simulink library "veh_vehicle_model_lib"  (R2016b)
settings: Solver=ode45  StartTime=0.0  StopTime=10.0  RelTol=1e-3  EnableMultiTasking=on
undefined symbols (not defined in the file): abp_impeller_speed2pwm, tun_sim_cg_error
libraries: util_generic_model_lib x2, epson_imu_model_lib x1
settings Model: Creator=jfusco1  LastModifiedBy=jfusco1
settings DataIOCC: LimitDataPoints=on  SaveFormat=Array
settings OptimizationCC: LifeSpan=inf
settings DebuggingCC: SolverPrmCheckMsg=warning  AllowSymbolicDim=off  SFUnexpectedBacktrackingDiag=warning  SFNoUnconditionalDefaultTransitionDiag=warning  SFExecutionAtInitializationDiag=none
settings HardwareCC: ProdBitPerPointer=32  ProdBitPerSizeT=32  ProdBitPerPtrDiffT=32  ProdLargestAtomicFloat=None  ProdIntDivRoundTo=Undefined  ProdEndianess=Unspecified  ProdWordSize=32  ProdHWDeviceType=32-bit Generic
settings ModelReferenceCC: PropagateSignalLabelsOutOfModel=off
settings GRTTargetCC: TargetLangStandard=C89/C90 (ANSI)  GeneratePreprocessorConditionals=Disable all
settings ConfigComp: CovMetricSettings=dw  CovHtmlReporting=on  CovSaveCumulativeToWorkspaceVar=on  CovSaveSingleToWorkspaceVar=on  CovExternalEMLEnable=off  CovSFcnEnable=off

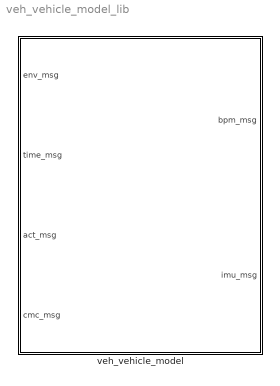
== system veh_vehicle_model_lib ==
  veh_vehicle_model : Subsystem

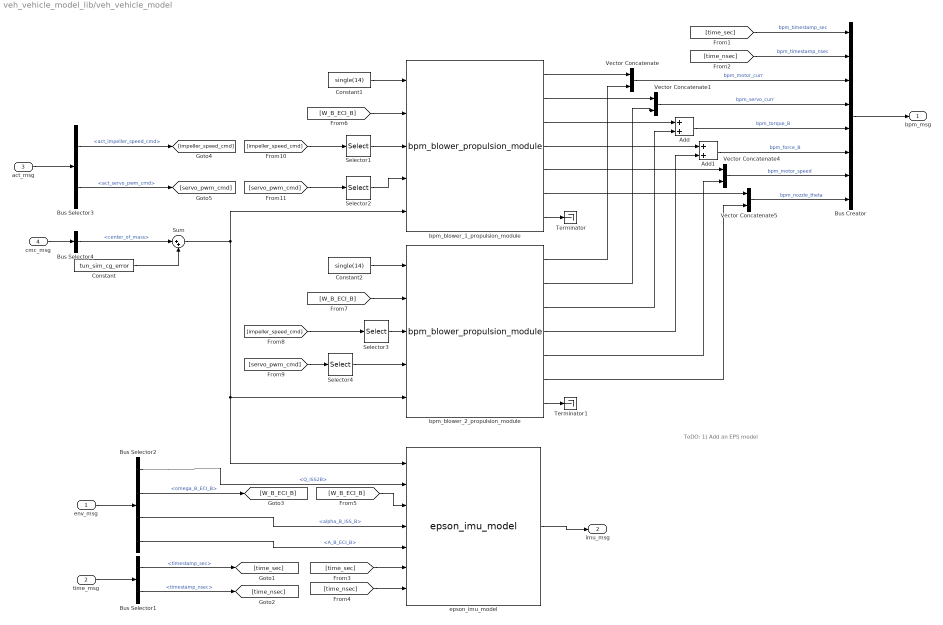
== system veh_vehicle_model_lib/veh_vehicle_model ==
  note: ToDO:
      | 1) Add an EPS model
  env_msg : Inport  OutDataTypeStr=Bus: env_msg
  time_msg : Inport  Port=2
  act_msg : Inport  Port=3
  cmc_msg : Inport  Port=4  OutDataTypeStr=Bus: cmc_msg
  Add : Sum
  Add1 : Sum
  Bus Creator : BusCreator  Inputs=8  OutDataTypeStr=Bus: bpm_msg  NonVirtualBus=on
      settings: InheritFromInputs=off
  Bus Selector1 : BusSelector  OutputSignals=timestamp_sec,timestamp_nsec
  Bus Selector2 : BusSelector  OutputSignals=Q_ISS2B,omega_B_ECI_B,alpha_B_ISS_B,A_B_ECI_B
  Bus Selector3 : BusSelector  OutputSignals=act_impeller_speed_cmd,act_servo_pwm_cmd
  Bus Selector4 : BusSelector  OutputSignals=center_of_mass
  Constant : Constant  Value=tun_sim_cg_error
  Constant1 : Constant  Value=single(14)
  Constant2 : Constant  Value=single(14)
  Selector1 : Selector  InputPortWidth=2  IndexOptions=Index vector (dialog)  Indices=1  OutputSizes=1
      settings: AttributesFormatString=|
      | Input Width: %<InputPortWidth>
      | Selection: %<Indices>
  Selector2 : Selector  InputPortWidth=12  IndexOptions=Index vector (dialog)  Indices=1:6  OutputSizes=1
      settings: AttributesFormatString=|
      | Input Width: %<InputPortWidth>
      | Selection: %<Indices>
  Selector3 : Selector  InputPortWidth=2  IndexOptions=Index vector (dialog)  Indices=2  OutputSizes=1
      settings: AttributesFormatString=|
      | Input Width: %<InputPortWidth>
      | Selection: %<Indices>
  Selector4 : Selector  InputPortWidth=12  IndexOptions=Index vector (dialog)  Indices=7:12  OutputSizes=1
      settings: AttributesFormatString=|
      | Input Width: %<InputPortWidth>
      | Selection: %<Indices>
  Sum : Sum  Inputs=|++
  Terminator : Terminator
  Terminator1 : Terminator
  Vector Concatenate{,1,4..5} (4 alike) : Concatenate
  bpm_blower_1_propulsion_module : util_generic_model_lib/bpm_blower_propulsion_module  s_ctl_ts=bpm_servo_ctl_ts  s_ctl_pwm2angle=bpm_servo_pwm2angle  s_ctl_pwm2angle_bias=bpm_servo_pwm2angle_bias  s_ctl_kp=bpm_servo_ctl_kp  s_ctl_ki=bpm_servo_ctl_ki  s_ctl_kd=bpm_servo_ctl_kd  s_ctl_filt_n=bpm_servo_ctl_filt_n  s_ctl_max_volt=bpm_servo_max_voltage  s_motor_k=bpm_servo_motor_k  s_motor_r=bpm_servo_motor_r  s_motor_friction_coeff=bpm_servo_motor_friction_coeff  s_motor_gear_ratio=bpm_servo_motor_gear_ratio  s_motor_gear_box_inertia=bpm_servo_motor_gear_box_inertia  servo_max_theta=bpm_servo_max_theta  servo_min_theta=bpm_servo_min_theta  servo_backlash_deadband=bpm_servo_motor_backlash_deadband  P_nozzle_B_B=abp_PM1_P_nozzle_B_B  P_nozzle_B_B_offset=bpm_PM1_P_nozzle_B_B_error  nozzle_orientation_B=abp_PM1_nozzle_orientations  nozzle_orientation_offset=bpm_PM1_Q_nozzle2misaligned  noz_cd=abp_PM1_discharge_coeff  noz_cd_error=bpm_PM1_nozzle_discharge_coeff_error  noz_width=abp_PM1_nozzle_widths  noz_min_theta=abp_nozzle_min_open_angle  noz_intake_height=abp_nozzle_intake_height  noz_flap_length=abp_nozzle_flap_length  noz_flap_count=abp_nozzle_flap_count  noz_gear_ratio=abp_nozzle_gear_ratio  noz_thrust_noise=bpm_PM1_nozzle_thrust_noise_1s  noz_thrust_noise_feedback=bpm_PM1_nozzle_noise_feedback_gain  noz_randn_seed=bpm_PM1_randn_noise_seed  i_ctl_ts=bpm_imp_ctl_ts  i_ctl_pwm2speed=1/abp_impeller_speed2pwm  i_ctl_cmd_filt_num=bpm_imp_cmd_filt_num  i_ctl_cmd_filt_den=bpm_imp_cmd_filt_den  i_ctl_speed_filt_num=bpm_imp_speed_filt_num  i_ctl_speed_filt_den=bpm_imp_speed_filt_den  i_ctl_kp=bpm_imp_ctl_kp  i_ctl_ki=bpm_imp_ctl_ki  i_ctl_kd=bpm_imp_ctl_kd  i_ctl_filt_n=bpm_imp_ctl_filt_n  i_ctl_max_volt=bpm_imp_max_voltage  i_motor_kn=bpm_imp_motor_speed_k  i_motor_r=bpm_imp_motor_r  i_motor_kt=bpm_imp_motor_torque_k  i_motor_friction_coeff=bpm_imp_motor_friction_coeff  imp_unit_vec_B=abp_pm1_impeller_orientation  imp_unit_vec_B_offset=bmp_PM1_impeller_orientation_error  imp_zero_thrust_area=abp_pm1_zero_thrust_area  imp_zero_thrust_area_error=bpm_PM1_zero_thrust_area_error  imp_diameter=abp_impeller_diameter  imp_cdp_lookup=bpm_lookup_Cdp_data  imp_area_lookup=bpm_lookup_totalarea_breakpoints  imp_inertia=bpm_impeller_inertia  imp_inertia_error=bpm_impeller_inertia_error  imp_init_speed=bpm_impeller_init_speed  sens_sf=bpm_sensor_sf  sens_sigma_u=bpm_sensor_sigma_u  sens_sigma_v=bpm_sensor_sigma_v  sens_rand_seed=bpm_sensor_rand_seed  sens_resolution=bpm_sensor_resolution  sens_max=bpm_sensor_max  sens_min=bpm_sensor_min  sens_delay=bpm_sensor_delay  P_CG_B_B_error=abp_P_CG_B_B_error  const_air_den=const_air_density  sim_step_size=astrobee_time_step_size  noise_on_flag=tun_bpm_noise_on_flag
  bpm_blower_2_propulsion_module : util_generic_model_lib/bpm_blower_propulsion_module  s_ctl_ts=bpm_servo_ctl_ts  s_ctl_pwm2angle=bpm_servo_pwm2angle  s_ctl_pwm2angle_bias=bpm_servo_pwm2angle_bias  s_ctl_kp=bpm_servo_ctl_kp  s_ctl_ki=bpm_servo_ctl_ki  s_ctl_kd=bpm_servo_ctl_kd  s_ctl_filt_n=bpm_servo_ctl_filt_n  s_ctl_max_volt=bpm_servo_max_voltage  s_motor_k=bpm_servo_motor_k  s_motor_r=bpm_servo_motor_r  s_motor_friction_coeff=bpm_servo_motor_friction_coeff  s_motor_gear_ratio=bpm_servo_motor_gear_ratio  s_motor_gear_box_inertia=bpm_servo_motor_gear_box_inertia  servo_max_theta=bpm_servo_max_theta  servo_min_theta=bpm_servo_min_theta  servo_backlash_deadband=bpm_servo_motor_backlash_deadband  P_nozzle_B_B=abp_PM2_P_nozzle_B_B  P_nozzle_B_B_offset=bpm_PM2_P_nozzle_B_B_error  nozzle_orientation_B=abp_PM2_nozzle_orientations  nozzle_orientation_offset=bpm_PM2_Q_nozzle2misaligned  noz_cd=abp_PM2_discharge_coeff  noz_cd_error=bpm_PM2_nozzle_discharge_coeff_error  noz_width=abp_PM2_nozzle_widths  noz_min_theta=abp_nozzle_min_open_angle  noz_intake_height=abp_nozzle_intake_height  noz_flap_length=abp_nozzle_flap_length  noz_flap_count=abp_nozzle_flap_count  noz_gear_ratio=abp_nozzle_gear_ratio  noz_thrust_noise=bpm_PM2_nozzle_thrust_noise_1s  noz_thrust_noise_feedback=bpm_PM2_nozzle_noise_feedback_gain  noz_randn_seed=bpm_PM2_randn_noise_seed  i_ctl_ts=bpm_imp_ctl_ts  i_ctl_pwm2speed=1/abp_impeller_speed2pwm  i_ctl_cmd_filt_num=bpm_imp_cmd_filt_num  i_ctl_cmd_filt_den=bpm_imp_cmd_filt_den  i_ctl_speed_filt_num=bpm_imp_speed_filt_num  i_ctl_speed_filt_den=bpm_imp_speed_filt_den  i_ctl_kp=bpm_imp_ctl_kp  i_ctl_ki=bpm_imp_ctl_ki  i_ctl_kd=bpm_imp_ctl_kd  i_ctl_filt_n=bpm_imp_ctl_filt_n  i_ctl_max_volt=bpm_imp_max_voltage  i_motor_kn=bpm_imp_motor_speed_k  i_motor_r=bpm_imp_motor_r  i_motor_kt=bpm_imp_motor_torque_k  i_motor_friction_coeff=bpm_imp_motor_friction_coeff  imp_unit_vec_B=abp_pm2_impeller_orientation  imp_unit_vec_B_offset=bmp_PM2_impeller_orientation_error  imp_zero_thrust_area=abp_pm2_zero_thrust_area  imp_zero_thrust_area_error=bpm_PM2_zero_thrust_area_error  imp_diameter=abp_impeller_diameter  imp_cdp_lookup=bpm_lookup_Cdp_data  imp_area_lookup=bpm_lookup_totalarea_breakpoints  imp_inertia=bpm_impeller_inertia  imp_inertia_error=bpm_impeller_inertia_error  imp_init_speed=bpm_impeller_init_speed  sens_sf=bpm_sensor_sf  sens_sigma_u=bpm_sensor_sigma_u  sens_sigma_v=bpm_sensor_sigma_v  sens_rand_seed=bpm_sensor_rand_seed  sens_resolution=bpm_sensor_resolution  sens_max=bpm_sensor_max  sens_min=bpm_sensor_min  sens_delay=bpm_sensor_delay  P_CG_B_B_error=abp_P_CG_B_B_error  const_air_den=const_air_density  sim_step_size=astrobee_time_step_size  noise_on_flag=tun_bpm_noise_on_flag
  epson_imu_model : epson_imu_model_lib/epson_imu_model
  bpm_msg : Outport
  imu_msg : Outport  Port=2
  wires:
  Selector4/1 -> bpm_blower_2_propulsion_module/4
  Selector3/1 -> bpm_blower_2_propulsion_module/3
  Selector2/1 -> bpm_blower_1_propulsion_module/4
  Selector1/1 -> bpm_blower_1_propulsion_module/3
  epson_imu_model/1 -> imu_msg/1
  env_msg/1 -> Bus Selector2/1
  Bus Selector2/2 -> [W_B_ECI_B]  "<omega_B_ECI_B>"
  Bus Selector3/2 -> [servo_pwm_cmd]  "<act_servo_pwm_cmd>"
  Bus Selector3/1 -> [impeller_speed_cmd]  "<act_impeller_speed_cmd>"
  act_msg/1 -> Bus Selector3/1
  time_msg/1 -> Bus Selector1/1
  Bus Selector1/2 -> [time_nsec]  "<timestamp_nsec>"
  Bus Selector1/1 -> [time_sec]  "<timestamp_sec>"
  [time_sec] -> Bus Creator/1  "bpm_timestamp_sec"
  [time_nsec] -> Bus Creator/2  "bpm_timestamp_nsec"
  Vector Concatenate5/1 -> Bus Creator/8  "bpm_nozzle_theta"
  Vector Concatenate4/1 -> Bus Creator/7  "bpm_motor_speed"
  Add/1 -> Bus Creator/5  "bpm_torque_B"
  Add1/1 -> Bus Creator/6  "bpm_force_B"
  Vector Concatenate1/1 -> Bus Creator/4  "bpm_servo_curr"
  Vector Concatenate/1 -> Bus Creator/3  "bpm_motor_curr"
  Bus Creator/1 -> bpm_msg/1
  Constant1/1 -> bpm_blower_1_propulsion_module/1
  Constant2/1 -> bpm_blower_2_propulsion_module/1
  [W_B_ECI_B] -> bpm_blower_1_propulsion_module/2
  [W_B_ECI_B] -> bpm_blower_2_propulsion_module/2
  [servo_pwm_cmd] -> Selector4/1
  [impeller_speed_cmd] -> Selector3/1
  [servo_pwm_cmd] -> Selector2/1
  [impeller_speed_cmd] -> Selector1/1
  bpm_blower_1_propulsion_module/1 -> Vector Concatenate/1
  bpm_blower_1_propulsion_module/2 -> Vector Concatenate1/1
  bpm_blower_1_propulsion_module/3 -> Add/1
  bpm_blower_1_propulsion_module/4 -> Add1/1
  bpm_blower_1_propulsion_module/5 -> Vector Concatenate4/1
  bpm_blower_1_propulsion_module/6 -> Vector Concatenate5/1
  bpm_blower_2_propulsion_module/1 -> Vector Concatenate/2
  bpm_blower_1_propulsion_module/7 -> Terminator/1
  bpm_blower_2_propulsion_module/7 -> Terminator1/1
  bpm_blower_2_propulsion_module/2 -> Vector Concatenate1/2
  bpm_blower_2_propulsion_module/3 -> Add/2
  bpm_blower_2_propulsion_module/4 -> Add1/2
  bpm_blower_2_propulsion_module/5 -> Vector Concatenate4/2
  bpm_blower_2_propulsion_module/6 -> Vector Concatenate5/2
  [W_B_ECI_B] -> epson_imu_model/3
  Bus Selector2/3 -> epson_imu_model/4  "<alpha_B_ISS_B>"
  Bus Selector2/4 -> epson_imu_model/5  "<A_B_ECI_B>"
  [time_sec] -> epson_imu_model/6
  [time_nsec] -> epson_imu_model/7
  Bus Selector2/1 -> epson_imu_model/2  "<Q_ISS2B>"
  cmc_msg/1 -> Bus Selector4/1
  Sum/1 -> epson_imu_model/1, bpm_blower_2_propulsion_module/5, bpm_blower_1_propulsion_module/5
  Bus Selector4/1 -> Sum/1  "<center_of_mass>"
  Constant/1 -> Sum/2
